simulink model "StarterSystemP2"  (R2020a)
settings: Solver=VariableStepAuto  StartTime=0.0  StopTime=inf  RelTol=1e-3
model workspace (MAT data in the model file):
  Iafser = 0
  Lafser = 0.01
  Lser = 0.06
  Plimit = 5000
  Rser = 0.1
  Tc = 0.001
  Vinit = 24
  VoltCmd = 24
  eff = 98
libraries: autolibdcdc x1, autolibstarter x1
settings Model: ModifiedByFormat=The MathWorks, Inc.  Creator=The MathWorks, Inc.  LastModifiedBy=The MathWorks, Inc.
settings SolverCC: AutoInsertRateTranBlk=on  DecoupledContinuousIntegration=on
settings DataIOCC: ReturnWorkspaceOutputs=off
settings DebuggingCC: PregeneratedLibrarySubsystemCodeDiagnostic=none  ArithmeticOperatorsInVariantConditions=warning
settings SFSimCC: SimUseLocalCustomCode=off  CustomCodeUndefinedFunction=UseInterfaceOnly
settings RTWCC: RTWUseLocalCustomCode=off

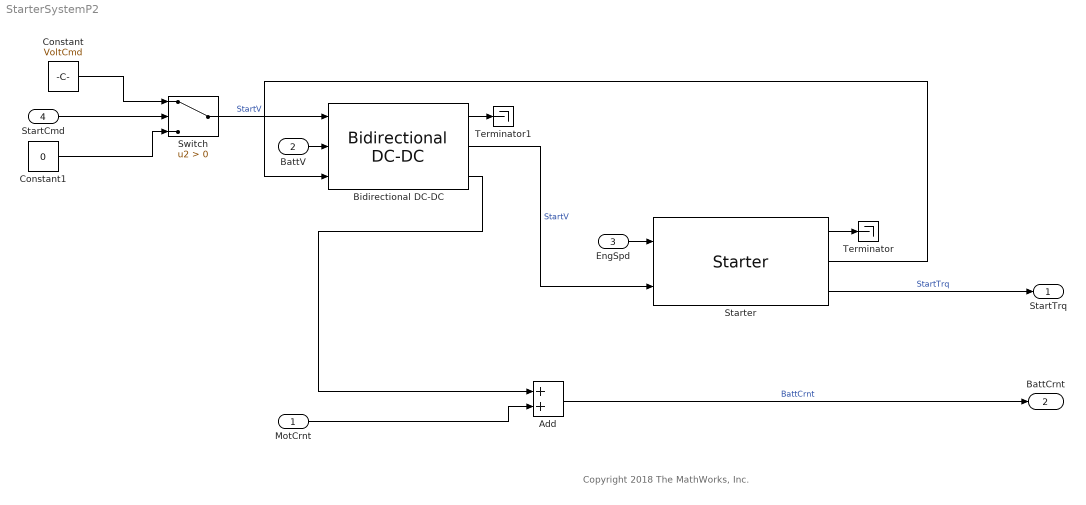
== system StarterSystemP2 ==
  note: Copyright 2018 The MathWorks, Inc.
  MotCrnt : Inport
  BattV : Inport  Port=2
  EngSpd : Inport  Port=3
  StartCmd : Inport  Port=4
  Add : Sum
  Bidirectional DC-DC : autolibdcdc/Bidirectional DC-DC  Tc=Tc  Vinit=Vinit  Plimit=Plimit  param_loss=Single efficiency measurement  eff=eff  v_loss_bp=[0 200 400 600 800 1000]  i_loss_bp=[0 25 50 75 100]  losses_table=[100 100 100 100 100;100 150 200 250 300;100 200 300 400 500;100 250 400 550 700;100 300 500 700 900;100 350 600 850 1100]  v_eff_bp=[200 400 600 800 1000]  i_eff_bp=[25 50 75 100]  efficiency_table=[96.2 98.1 98.7 99;98.1 99 99.4 99.5;98.7 99.4 99.6 99.7;99 99.5 99.7 99.8;99.2 99.6 99.7 99.8]  x_v_bp=[-1000 -800 -600 -400 -200 200 400 600 800 1000]  x_i_bp=[-100 -75 -50 -25 25 50 75 100]  x_losses_mat=[200.400801603196 225.67703109328 200.803212851408 201.612903225806 199.999999999997 200 225 200;160.320641282556 180.541624874624 201.005025125625 202.020202020203 200 200 180 160;180.541624874624 180.722891566267 181.086519114686 197.568389057748 194.999999999999 179.999999999997 180 180;201.005025125625 181.086519114686 202.020202020203 193.67991845056 190 200 179.999999999997 200;202.020202020203 197.568389057748 193.67991845056 197.505197505197 190 190 194.999999999999 200;200 194.999999999999 190 190 197.505197505197 193.67991845056 197.568389057748 202.020202020203;200 179.999999999997 200 190 193.67991845056 202.020202020203 181.086519114686 201.005025125625;180 180 179.999999999997 194.999999999999 197.568389057748 181.086519114686 180.722891566267 180.541624874624;160 180 200 200 202.020202020203 201.005025125625 180.541624874624 160.320641282556;200 225 200 199.999999999997 201.612903225806 200.803212851408 225.67703109328 200.400801603196]  RefBlkName='autolibdcdc/Bidirectional DC-DC'
      settings: SourceProductBaseCode=PW
  Constant : Constant  Value=VoltCmd
  Constant1 : Constant  Value=0
  Starter : autolibstarter/Starter  machine_type=Series Connection DC Motor  Ra=1  La=.1  Rf=.3  Lf=.2  Laf=.3  Iaf=[0 0]  Rapm=0.03  Lapm=0.000042  Kt=0.1  Ia=0  Rser=Rser  Lser=Lser  Iafser=Iafser  Lafser=Lafser  RefBlkName='autolibstarter/Starter'
      settings: SourceProductBaseCode=PW
  Switch : Switch  Criteria=u2 > Threshold
  Terminator : Terminator
  Terminator1 : Terminator
  StartTrq : Outport  VectorParamsAs1DForOutWhenUnconnected=off
  BattCrnt : Outport  Port=2  VectorParamsAs1DForOutWhenUnconnected=off
  wires:
  Bidirectional DC-DC/1 -> Terminator1/1
  Starter/3 -> StartTrq/1  "StartTrq"
  Add/1 -> BattCrnt/1  "BattCrnt"
  MotCrnt/1 -> Add/2
  StartCmd/1 -> Switch/2
  Bidirectional DC-DC/2 -> Starter/2  "StartV"
  Bidirectional DC-DC/3 -> Add/1
  Starter/2 -> Bidirectional DC-DC/3
  Constant1/1 -> Switch/3
  EngSpd/1 -> Starter/1
  Starter/1 -> Terminator/1
  Constant/1 -> Switch/1
  BattV/1 -> Bidirectional DC-DC/2
  Switch/1 -> Bidirectional DC-DC/1  "StartV"
